simulink model "SyncGenSim"  (R2013a)
settings: Solver=ode45  StartTime=5  StopTime=10  FixedStep=10^-3  MaxStep=10^-2  RelTol=1e-2
undefined symbols (not defined in the file): J, R_l, T_m, V_f
libraries: powerlib x6, powerlib_meascontrol x1, SyncGenLib x1
settings Model: Creator=Elad  LastModifiedBy=USER
settings DataIOCC: SignalLoggingSaveFormat=ModelDataLogs
settings DebuggingCC: MultiTaskDSMMsg=warning  MultiTaskCondExecSysMsg=none  StateNameClashWarn=none  StrictBusMsg=None
settings RTWCC: IncludeERTFirstTime=on

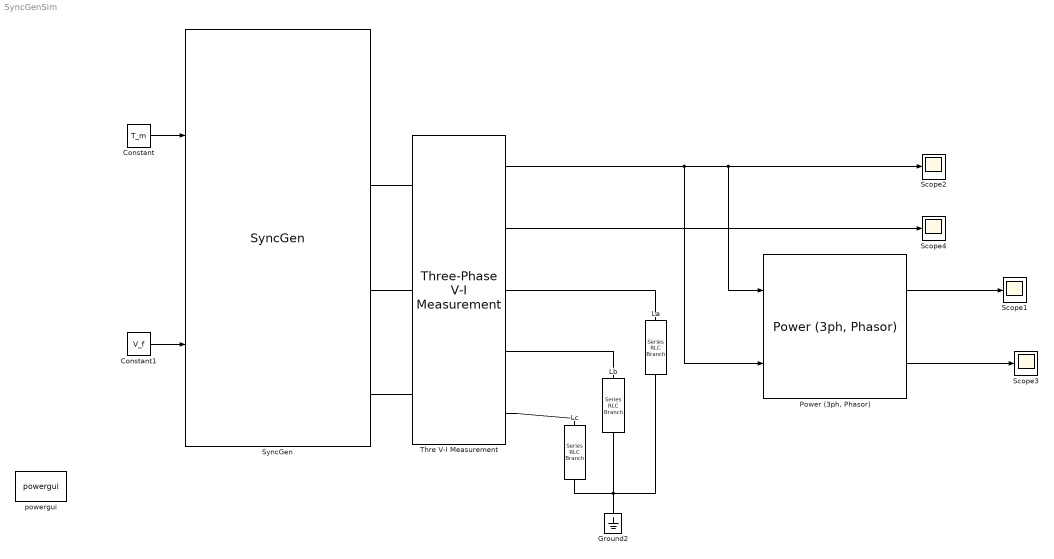
== system SyncGenSim ==
  " Lb " : powerlib/Elements/Series RLC Branch  LConnTagsString=__new0  RConnTagsString=__new0  BranchType=R  Resistance=R_l  Inductance=1e-3  SetiL0=off  InitialCurrent=0  Capacitance=1e-6  Setx0=off  InitialVoltage=0  Measurements=None
  Constant : Constant  Value=T_m
  Constant1 : Constant  Value=V_f
  Ground2 : powerlib/Elements/Ground  LConnTagsString=a
  La : powerlib/Elements/Series RLC Branch  LConnTagsString=__new0  RConnTagsString=__new0  BranchType=R  Resistance=R_l  Inductance=1e-3  SetiL0=off  InitialCurrent=0  Capacitance=1e-6  Setx0=off  InitialVoltage=0  Measurements=None
  "Lc  " : powerlib/Elements/Series RLC Branch  LConnTagsString=__new0  RConnTagsString=__new0  BranchType=R  Resistance=R_l  Inductance=1e-3  SetiL0=off  InitialCurrent=0  Capacitance=1e-6  Setx0=off  InitialVoltage=0  Measurements=None
  "Power (3ph, Phasor)" : powerlib_meascontrol/Measurements/Power (3ph, Phasor)
  Scope{1..4} (4 alike) : Scope
      Scope1 settings: TimeRange=5  YMin=3.95e+06  YMax=4.16e+06
      Scope2 settings: TimeRange=5  YMin=-2500  YMax=2500
      Scope3 settings: TimeRange=5  YMin=-225  YMax=225  SaveName=ScopeData3
      Scope4 settings: TimeRange=5  YMin=-0.5  YMax=0.5  SaveName=ScopeData4
  "SyncGen " : SyncGenLib/SyncGen   R_f=R_f  R_s=R_f  D_p=D_p  J=J  M_f=M_f  L_f=L_f  L_s=L_s
  Thre V-I Measurement : powerlib/Measurements/Three-Phase V-I Measurement  VoltageMeasurement=phase-to-ground  SetLabelV=off  LabelV=Vabc  Vpu=off  VpuLL=off  CurrentMeasurement=yes  SetLabelI=off  LabelI=Iabc  Ipu=off  Pbase=100e6  Vbase=500e3  OutputType=Complex  PhasorSimulation=off  PSBequivalent=0
  powergui : powerlib/powergui  Priority=1  SimulationMode=Continuous  SolverType=Tustin  SampleTime=50e-6  frequency=60  SPID=off  DisableSnubberDevices=off  DisableRonSwitches=off  DisableVfSwitches=off  SwTol=0  Interpol=off  DisplayEquations=off  frequencyindice=0  Pbase=100e6  ErrMax=1e-4  Iterations=50  UnitsV=kV  UnitsW=MW  FunctionMessages=off  echomessages=off  HookPort=off  EnableUseOfTLC=off  x0status=blocks  RestoreLinks=warning  ResistiveCurrentMeasurement=off  Frange=[0:2:500]  Ylog=off  Xlog=on  ShowGrid=off  save=off  variable=ZData  ZoomFFT=off  StartTime=0.0  cycles=1  DisplayStyle=1  fundamental=60  FreqAxis=off  MaxFrequency=1000  frequencyindicesteady=1  RmsSteady=1  display=off  Ts=0  methode=off
  wires:
  "Power (3ph, Phasor)"/1 -> Scope1/1
  "Power (3ph, Phasor)"/2 -> Scope3/1
  Thre V-I Measurement/1 -> "Power (3ph, Phasor)"/2, "Power (3ph, Phasor)"/1, Scope2/1
  Thre V-I Measurement/2 -> Scope4/1
  Constant/1 -> "SyncGen "/1
  Constant1/1 -> "SyncGen "/2
  connections:
  "Lc  "/RConn1 -- La/RConn1 -- Ground2/LConn1 -- " Lb "/RConn1
  "SyncGen "/RConn1 -- Thre V-I Measurement/LConn1
  "SyncGen "/RConn2 -- Thre V-I Measurement/LConn2
  "SyncGen "/RConn3 -- Thre V-I Measurement/LConn3
  Thre V-I Measurement/RConn3 -- "Lc  "/LConn1
  Thre V-I Measurement/RConn2 -- " Lb "/LConn1
  Thre V-I Measurement/RConn1 -- La/LConn1
